simulink model "Test_Tricopter_Model"  (R2015a)
settings: Solver=ode3  SolverMode=SingleTasking  StartTime=0.0  StopTime=20  FixedStep=T_sim  RelTol=1e-3
PreLoadFcn:
  | LoadLibraries
values from neighbouring files (symbols this model uses):
  a = 10.26    [SetupComplete.m]
  A_x = 0.015    [SetupComplete.m]
  A_y = A_x    (= 0.015)    [SetupComplete.m]
  A_z = 0.16    [SetupComplete.m]
  C_d0 = 0.001193    [SetupComplete.m]
  C_x = 1.2    [SetupComplete.m]
  C_y = C_x    (= 1.2)    [SetupComplete.m]
  C_z = 2.2    [SetupComplete.m]
  CG_0 = [0,0,0.02]'    [SetupComplete.m]
  g = 9.81    [SetupComplete.m]
  h = 0.08    [SetupComplete.m]
  h_FA = 0.02    [SetupComplete.m]
  h_M = 0.064    [SetupComplete.m]
  I_BAC_0 = [ Ix,0,Ixz;0,Iy,0;Ixz,0,Iz]    [SetupComplete.m]
  I_prop = 1/4*M_eq*R^2*diag([1,1,2])    [SetupComplete.m]
  I_tube = [1/2*M_tube*R_tube_eq^2,0,  0  ;           0 ,1/3*M_tube*l_arm^2,0;             0  ,0,1/3*M_tube*l_arm^2]    [SetupComplete.m]
  Initial_Omegas = [1;1;1]*Omega_hover    [Run3Copter.m]
  J_FA = I_prop(1,1) + m_prop*h^2  + m_FA*h_FA^2 + m_M*h_M^2    [SetupComplete.m]
  J_T = J_m+1/2*M_eq*R^2    (= 2.000642e-05)    [SetupComplete.m]
  Ki = lqi(LM_4DOF_aug, Q,R)    [robust_controller.m]
  l = 0.3450    (= 0.345)    [NDI_components.m]    (also in SetupComplete.m; robust_controller.m)
  l_arm = 0.264    [SetupComplete.m]
  m = 3.51    [SetupComplete.m]
  m_0 = 2.61    [SetupComplete.m]
  m_FA = 0.02    [SetupComplete.m]
  m_M = 0.300    (= 0.3)    [SetupComplete.m]
  m_prop = 0.02    [SetupComplete.m]
  R = 0.1778    [SetupComplete.m]    (also in robust_controller.m = eye(4))
  rho = 1.15    [SetupComplete.m]
  sigma = b*c/(pi*R)    (= 0.107416159567)    [SetupComplete.m]
  T_sim = 0.01    [Run3Copter.m]
  theta_0 = 0.38397    [SetupComplete.m]
  theta_1 = -0.2967    [SetupComplete.m]
  trim_simplemodel = [0.589627915568 -2.20656039197 0 0.588313336084 0 0 0.588313330414 0 0]    [trimvalues.mat]
  V_4DOF_last = [0.0122475086001 0.00870447045314 -0.0292257707267 -0.0198753669721 -0.00290766514824 -0.0269511839788 0.0344308792695 -0.0305235710433 -0.0274078219028 -0.0329291952852 -0.0272335702183 -0.00643013158961 ... (1500 elements, 50x30)]    [NN_c_weights.mat]
  v_i0 = sqrt( 1/3*m*g/(2*rho*pi*R^2)  )    [SetupComplete.m]
  W_4DOF_last = [0.0132359246225 -0.0402459595001 -0.0221501781133 0.0046881519205 0.0457506835434 0.0464888535199 -0.0342386918322 0.0470592781761 0.0457166948243 -0.00146243512772 0.0300280468889 -0.0358113661373 ... (204 elements, 4x51)]    [NN_c_weights.mat]
undefined symbols (not defined in the file or in its folder): DOWN_0, EAST_0, Motor, NORTH_0, P_0, Prop, Q_0, R_0, sigmatest, U_0, V_0, v_i_adim, Vx_adim, Vz_adim, W_0
undefined symbols (not defined in the file): Initial_Torques, Rotation_sign, Tau_motors
libraries: simulink x61, XXCopter x32, vrlib x26, simulink_extras x6, aerolib6dofsys x3, qcatlib x3, dspinverses x3, lib_controller x2, aerolibtransform2 x2, aerolib6dof2 x1
(part 4 of 10)

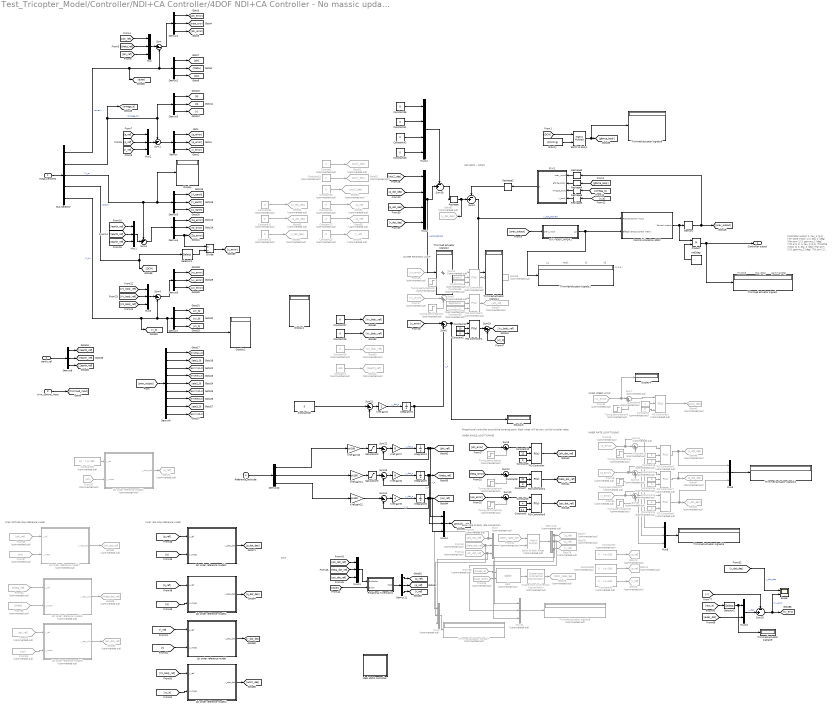
== system Test_Tricopter_Model/Controller/NDI+CA Controller/4DOF NDI+CA Controller - No massic update ==
  note: 16 8
  note: Inner rate loop reference model
  note: w
      | p
      | q
      | r
  note: t1
  note: t2
  note: t3
  note: eta1
  note: OUTER POSITION LOOP
  note: gamma[deg]
  note: eta [deg]
  note: Throttle
  note: Controller output:
      | 1. tau_1 [0-1] (Thr ottle motor 1)
      | 2. eta_1 (deg)  (Pan arm 1)
      | 3. gamma_1 (deg)  (Tilt arm 1)
      |
      | 4. tau_2 [0-1] (Throttle motor 2)
      | 5. eta_2 (deg)  (Pan arm 2)
      | 6. gamma_2 (deg)  (Tilt arm 2)
      |
      | 7. tau_3 [0-1] (Throttle motor 3)
      | 8. eta_3 (deg)  (Pan arm  3)
      | 9. gamma_3 (deg)  (Tilt arm 3)
  note: Proportional controller around the hovering point. Body rates will be very similar to euler rates.
  note: INNER RATE LOOP TUNING
  note: INNER ANGLE LOOP TUNING
  note: INNER SPEED LOOP
  note: NDI 4DOF - WPQR
  note: Euler rate to body rate conversion
  note: Inner attitude loop reference model
  measurements : Inport
  earth_ref : Inport  Port=2
  trim_control_input : Inport  Port=3
  Reference_attitude : Inport  Port=4
  1st order reference model : Subsystem  mask(1st order model reference block){Kref=10, Kb=10, fi=0.25, fc=0.5, Kf=1}
      mask prompts: Kref "1st order reference gain"; Kb "Bandwidth gain"; fi "Integral gain"; fc "Command FF gain"; Kf "Command_dot FF gain"
      mask help:
      | Generates a desired first order derivative of a commanded output taking
      | into account the current measured output.
      | Kref is the gain that determines the first order system between y_ref and
      | y_commanded signals. Ycom/Yref = Kref/(1 + Kref)
      | fi and fc can be defaulted to 0.25 and 0.5 for a critically damped 2nd
      | order response between y_meas and the error signal (y_com - y_meas) considering
      | a perfect dynamic inversion.
      mask Help:
      | Juan Herrero Macias <jn.herrerom@gmail.com>
      | This architecture can be found and explained in Fault-tolerant Flight
      | Control and Guidance Systems, Ducard, Guillaume.
      mask TypeOptions Kref: Kref gain/Gain
      mask TypeOptions Kb: Bandwidth gain/Gain
      mask TypeOptions fi: Integral gain/Gain
      mask TypeOptions fc: Command FF gain/Gain
      mask TypeOptions Kf: Command_dot FF gain/Gain
  1st order reference model1 : Subsystem  mask(1st order model reference block){Kref=8, Kb=16, fi=0.25, fc=0.5, Kf=1}
      mask prompts: Kref "1st order reference gain"; Kb "Bandwidth gain"; fi "Integral gain"; fc "Command FF gain"; Kf "Command_dot FF gain"
      mask help:
      | Generates a desired first order derivative of a commanded output taking
      | into account the current measured output.
      | Kref is the gain that determines the first order system between y_ref and
      | y_commanded signals. Ycom/Yref = Kref/(1 + Kref)
      | fi and fc can be defaulted to 0.25 and 0.5 for a critically damped 2nd
      | order response between y_meas and the error signal (y_com - y_meas) considering
      | a perfect dynamic inversion.
      mask Help:
      | Juan Herrero Macias <jn.herrerom@gmail.com>
      | This architecture can be found and explained in Fault-tolerant Flight
      | Control and Guidance Systems, Ducard, Guillaume.
      mask TypeOptions Kref: Kref gain/Gain
      mask TypeOptions Kb: Bandwidth gain/Gain
      mask TypeOptions fi: Integral gain/Gain
      mask TypeOptions fc: Command FF gain/Gain
      mask TypeOptions Kf: Command_dot FF gain/Gain
  1st order reference model2 : Subsystem  mask(1st order model reference block){Kref=8, Kb=16, fi=0.25, fc=0.5, Kf=1}
      mask prompts: Kref "1st order reference gain"; Kb "Bandwidth gain"; fi "Integral gain"; fc "Command FF gain"; Kf "Command_dot FF gain"
      mask help:
      | Generates a desired first order derivative of a commanded output taking
      | into account the current measured output.
      | Kref is the gain that determines the first order system between y_ref and
      | y_commanded signals. Ycom/Yref = Kref/(1 + Kref)
      | fi and fc can be defaulted to 0.25 and 0.5 for a critically damped 2nd
      | order response between y_meas and the error signal (y_com - y_meas) considering
      | a perfect dynamic inversion.
      mask Help:
      | Juan Herrero Macias <jn.herrerom@gmail.com>
      | This architecture can be found and explained in Fault-tolerant Flight
      | Control and Guidance Systems, Ducard, Guillaume.
      mask TypeOptions Kref: Kref gain/Gain
      mask TypeOptions Kb: Bandwidth gain/Gain
      mask TypeOptions fi: Integral gain/Gain
      mask TypeOptions fc: Command FF gain/Gain
      mask TypeOptions Kf: Command_dot FF gain/Gain
  1st order reference model3 : Subsystem  Commented=on  mask(1st order model reference block){Kref=2, Kb=2, fi=0.25, fc=0, Kf=0}
      mask prompts: Kref "1st order reference gain"; Kb "Bandwidth gain"; fi "Integral gain"; fc "Command FF gain"; Kf "Command_dot FF gain"
      mask help:
      | Generates a desired first order derivative of a commanded output taking
      | into account the current measured output.
      | Kref is the gain that determines the first order system between y_ref and
      | y_commanded signals. Ycom/Yref = Kref/(1 + Kref)
      | fi and fc can be defaulted to 0.25 and 0.5 for a critically damped 2nd
      | order response between y_meas and the error signal (y_com - y_meas) considering
      | a perfect dynamic inversion.
      mask Help:
      | Juan Herrero Macias <jn.herrerom@gmail.com>
      | This architecture can be found and explained in Fault-tolerant Flight
      | Control and Guidance Systems, Ducard, Guillaume.
      mask TypeOptions Kref: Kref gain/Gain
      mask TypeOptions Kb: Bandwidth gain/Gain
      mask TypeOptions fi: Integral gain/Gain
      mask TypeOptions fc: Command FF gain/Gain
      mask TypeOptions Kf: Command_dot FF gain/Gain
  1st order reference model4 : Subsystem  mask(1st order model reference block){Kref=4, Kb=8, fi=0.25, fc=0.5, Kf=1}
      mask prompts: Kref "1st order reference gain"; Kb "Bandwidth gain"; fi "Integral gain"; fc "Command FF gain"; Kf "Command_dot FF gain"
      mask help:
      | Generates a desired first order derivative of a commanded output taking
      | into account the current measured output.
      | Kref is the gain that determines the first order system between y_ref and
      | y_commanded signals. Ycom/Yref = Kref/(1 + Kref)
      | fi and fc can be defaulted to 0.25 and 0.5 for a critically damped 2nd
      | order response between y_meas and the error signal (y_com - y_meas) considering
      | a perfect dynamic inversion.
      mask Help:
      | Juan Herrero Macias <jn.herrerom@gmail.com>
      | This architecture can be found and explained in Fault-tolerant Flight
      | Control and Guidance Systems, Ducard, Guillaume.
      mask TypeOptions Kref: Kref gain/Gain
      mask TypeOptions Kb: Bandwidth gain/Gain
      mask TypeOptions fi: Integral gain/Gain
      mask TypeOptions fc: Command FF gain/Gain
      mask TypeOptions Kf: Command_dot FF gain/Gain
  1st order reference model5 : Subsystem  Commented=on  mask(1st order model reference block){Kref=8, Kb=4, fi=0.25, fc=0.5, Kf=1}
      mask prompts: Kref "1st order reference gain"; Kb "Bandwidth gain"; fi "Integral gain"; fc "Command FF gain"; Kf "Command_dot FF gain"
      mask help:
      | Generates a desired first order derivative of a commanded output taking
      | into account the current measured output.
      | Kref is the gain that determines the first order system between y_ref and
      | y_commanded signals. Ycom/Yref = Kref/(1 + Kref)
      | fi and fc can be defaulted to 0.25 and 0.5 for a critically damped 2nd
      | order response between y_meas and the error signal (y_com - y_meas) considering
      | a perfect dynamic inversion.
      mask Help:
      | Juan Herrero Macias <jn.herrerom@gmail.com>
      | This architecture can be found and explained in Fault-tolerant Flight
      | Control and Guidance Systems, Ducard, Guillaume.
      mask TypeOptions Kref: Kref gain/Gain
      mask TypeOptions Kb: Bandwidth gain/Gain
      mask TypeOptions fi: Integral gain/Gain
      mask TypeOptions fc: Command FF gain/Gain
      mask TypeOptions Kf: Command_dot FF gain/Gain
  1st order reference model6 : Subsystem  Commented=on  mask(1st order model reference block){Kref=2, Kb=4, fi=0.25, fc=0.5, Kf=1}
      mask prompts: Kref "1st order reference gain"; Kb "Bandwidth gain"; fi "Integral gain"; fc "Command FF gain"; Kf "Command_dot FF gain"
      mask help:
      | Generates a desired first order derivative of a commanded output taking
      | into account the current measured output.
      | Kref is the gain that determines the first order system between y_ref and
      | y_commanded signals. Ycom/Yref = Kref/(1 + Kref)
      | fi and fc can be defaulted to 0.25 and 0.5 for a critically damped 2nd
      | order response between y_meas and the error signal (y_com - y_meas) considering
      | a perfect dynamic inversion.
      mask Help:
      | Juan Herrero Macias <jn.herrerom@gmail.com>
      | This architecture can be found and explained in Fault-tolerant Flight
      | Control and Guidance Systems, Ducard, Guillaume.
      mask TypeOptions Kref: Kref gain/Gain
      mask TypeOptions Kb: Bandwidth gain/Gain
      mask TypeOptions fi: Integral gain/Gain
      mask TypeOptions fc: Command FF gain/Gain
      mask TypeOptions Kf: Command_dot FF gain/Gain
  1st order reference model7 : Subsystem  Commented=on  mask(1st order model reference block){Kref=8, Kb=4, fi=0.25, fc=0.5, Kf=1}
      mask prompts: Kref "1st order reference gain"; Kb "Bandwidth gain"; fi "Integral gain"; fc "Command FF gain"; Kf "Command_dot FF gain"
      mask help:
      | Generates a desired first order derivative of a commanded output taking
      | into account the current measured output.
      | Kref is the gain that determines the first order system between y_ref and
      | y_commanded signals. Ycom/Yref = Kref/(1 + Kref)
      | fi and fc can be defaulted to 0.25 and 0.5 for a critically damped 2nd
      | order response between y_meas and the error signal (y_com - y_meas) considering
      | a perfect dynamic inversion.
      mask Help:
      | Juan Herrero Macias <jn.herrerom@gmail.com>
      | This architecture can be found and explained in Fault-tolerant Flight
      | Control and Guidance Systems, Ducard, Guillaume.
      mask TypeOptions Kref: Kref gain/Gain
      mask TypeOptions Kb: Bandwidth gain/Gain
      mask TypeOptions fi: Integral gain/Gain
      mask TypeOptions fc: Command FF gain/Gain
      mask TypeOptions Kf: Command_dot FF gain/Gain
  Bus Selector : BusSelector  OutputSignals=euler,omega_b,X_e,DCM,V_b
  Constant{,3,14,16,18..23,29..33,35} (16 alike) : Constant  Commented=on  Value=0
  Constant1 : Constant  Commented=on  Value=-100
  Constant10 : Constant  Value=12
  Constant11 : Constant  Value=10
  Constant12 : Constant  Commented=on  Value=deg2rad(1)
  Constant13 : Constant  Commented=on  Value=6
  Constant15 : Constant  Commented=on  Value=5
  Constant17 : Constant  Commented=on  Value=6
  Constant{2,27..28,36,41..43,45} (8 alike) : Constant  Value=0
  Constant34 : Constant  Commented=on  Value=deg2rad(1)
  Constant37 : Constant  Commented=on  Value="0     * pi /180"
  Constant38 : Constant  Commented=on  Value="10     * pi /180"
  Constant39 : Constant  Commented=on  Value="0     * pi /180"
  Constant4 : Constant  Commented=on
  Constant40 : Constant  Commented=on  Value="0     * pi /180"
  Constant5 : Constant  Value=0.4
  Constant6 : Constant  Value=4
  Constant7 : Constant  Value=3
  Constant8 : Constant  Value=12
  Constant9 : Constant  Value=3
  Control Allocation 4DOF : Subsystem  Variant=on  OverrideUsingVariant=Variant1
  Demux{,1..8,11,13} (11 alike) : Demux  Outputs=3
  Demux10 : Demux  Commented=on  Outputs=3
  Demux9 : Demux  Outputs=9
  Display{,1..4} (5 alike) : Display
  Divide : Product  Inputs=*/
  Earth to body Rates : Product  Commented=on  Multiplication=Matrix(*)
  Earth to body1 : Product  Multiplication=Matrix(*)
  F(X)1 : MATLAB Function  TreatAsAtomicUnit=on
  From17 : From  Commented=on  GotoTag=vy_error
  From18 : From  Commented=on  GotoTag=vx_error
  From21 : From  Commented=on  GotoTag=vz_error
  From25 : From  Commented=on  GotoTag=quat_euler
  From26 : From  Commented=on  GotoTag=p_error
  From28 : From  Commented=on  GotoTag=q_error
  From29 : From  Commented=on  GotoTag=r_error
  From35 : From  Commented=on  GotoTag=phi
  From36 : From  Commented=on  GotoTag=omega_b
  From37 : From  Commented=on  GotoTag=phi_dot_ref
  From40 : From  Commented=on  GotoTag=theta_dot_ref
  From41 : From  Commented=on  GotoTag=psi_dot_ref
  From42 : From  Commented=on  GotoTag=DCM_rates_be
  From54 : From  Commented=on  GotoTag=theta_ref
  From55 : From  Commented=on  GotoTag=theta
  From56 : From  Commented=on  GotoTag=phi_ref
  From57 : From  Commented=on  GotoTag=phi
  From58 : From  Commented=on  GotoTag=psi_ref
  From59 : From  Commented=on  GotoTag=psi
  G(X) 4DOF_WPQR1 : MATLAB Function  TreatAsAtomicUnit=on
  Goto40 : Goto  Commented=on  GotoTag=Zearth_ref
  Goto41 : Goto  Commented=on  GotoTag=accZ_des
  Goto46 : Goto  Commented=on  GotoTag=p_dot_des
  Goto47 : Goto  Commented=on  GotoTag=q_dot_des
  Goto48 : Goto  Commented=on  GotoTag=r_dot_des
  Goto51 : Goto  Commented=on  GotoTag=accX_des
  Goto52 : Goto  Commented=on  GotoTag=accY_des
  Goto53 : Goto  Commented=on  GotoTag=accZ_des
  Goto{54,72..73,77} (4 alike) : Goto  Commented=on  GotoTag=p_ref
  Goto55 : Goto  Commented=on  GotoTag=q_ref
  Goto56 : Goto  Commented=on  GotoTag=r_ref
  Goto63 : Goto  Commented=on  GotoTag=Vz_body_ref
  Goto64 : Goto  Commented=on  GotoTag=p_dot_des
  Goto65 : Goto  Commented=on  GotoTag=q_dot_des
  Goto66 : Goto  Commented=on  GotoTag=r_dot_des
  Goto67 : Goto  Commented=on  GotoTag=phi_ref
  Goto68 : Goto  Commented=on  GotoTag=theta_ref
  Goto74 : Goto  Commented=on  GotoTag=q_ref
  Goto75 : Goto  Commented=on  GotoTag=r_ref
  Goto76 : Goto  Commented=on  GotoTag=DCM_rates_be
  Goto78 : Goto  Commented=on  GotoTag=q_ref
  Goto79 : Goto  Commented=on  GotoTag=r_ref
  Goto87 : Goto  Commented=on  GotoTag=y_dot_des
  Goto89 : Goto  Commented=on  GotoTag=theta_dot_ref
  Goto90 : Goto  Commented=on  GotoTag=phi_dot_ref
  Goto91 : Goto  Commented=on  GotoTag=psi_dot_ref
  Gravity : Constant  Value=[0;0;m*g]
  Ideal 4DOF controller : Subsystem
  Integrator{3..6} (4 alike) : Integrator
  Kref gain10 : Gain  Gain=pi/180
  Kref gain11 : Gain  Gain=pi/180
  Kref gain12 : Gain  Gain=pi/180
  Kref gain3 : Gain
  Kref gain7 : Gain  Gain=6
  Kref gain8 : Gain  Gain=6
  Kref gain9 : Gain  Gain=4
  Memory : Memory  X0=[0,0,0,0,0,0,0,0,0]  LinearizeAsDelay=on
  Mux{,1..3,5,8,11,14} (8 alike) : Mux  Inputs=3
  Mux10 : Mux  Commented=on  Inputs=3
  Mux12 : Mux
  Mux13 : Mux  Inputs=2
  Mux4 : Mux
  Mux7 : Mux  Commented=on  Inputs=3
  Mux9 : Mux  Commented=on  Inputs=3
  PID Controller{,1,4..5} (4 alike) : simulink/Continuous/PID Controller  Controller=PI  TimeDomain=Continuous-time  SampleTime=-1  IntegratorMethod=Forward Euler  FilterMethod=Forward Euler  Form=Parallel  UseFilter=on  ControllerParametersSource=external  P=1  I=1  D=0  N=100  InitialConditionSource=internal  InitialConditionForIntegrator=0  InitialConditionForFilter=0  ExternalReset=none  LimitOutput=off  UpperSaturationLimit=inf  LowerSaturationLimit=-inf  LinearizeAsGain=on  AntiWindupMode=none  Kb=1  TrackingMode=off  Kt=1  PParamMin=[]  PParamMax=[]  IParamMin=[]  IParamMax=[]  DParamMin=[]  DParamMax=[]  NParamMin=[]  NParamMax=[]  KbParamMin=[]  KbParamMax=[]  KtParamMin=[]  KtParamMax=[]  POutMin=[]  POutMax=[]  IOutMin=[]  IOutMax=[]  DOutMin=[]  DOutMax=[]  NOutMin=[]  NOutMax=[]  KbOutMin=[]  KbOutMax=[]  KtOutMin=[]  KtOutMax=[]  IntegratorOutMin=[]  IntegratorOutMax=[]  FilterOutMin=[]  FilterOutMax=[]  SumOutMin=[]  SumOutMax=[]  SumI1OutMin=[]  SumI1OutMax=[]  SumI2OutMin=[]  SumI2OutMax=[]  SumI3OutMin=[]  SumI3OutMax=[]  SumDOutMin=[]  SumDOutMax=[]  SaturationOutMin=[]  SaturationOutMax=[]  IntegratorContinuousStateAttributes=''  IntegratorStateMustResolveToSignalObject=off  IntegratorRTWStateStorageClass=Auto  FilterContinuousStateAttributes=''  FilterStateMustResolveToSignalObject=off  FilterRTWStateStorageClass=Auto  DifferentiatorICPrevScaledInput=0  DifferentiatorOutMin=[]  DifferentiatorOutMax=[]
  PID Controller{2..3,8..9} (4 alike) : simulink/Continuous/PID Controller  Commented=on  Controller=PI  TimeDomain=Continuous-time  SampleTime=-1  IntegratorMethod=Forward Euler  FilterMethod=Forward Euler  Form=Parallel  UseFilter=on  ControllerParametersSource=external  P=1  I=1  D=0  N=100  InitialConditionSource=internal  InitialConditionForIntegrator=0  InitialConditionForFilter=0  ExternalReset=none  LimitOutput=off  UpperSaturationLimit=inf  LowerSaturationLimit=-inf  LinearizeAsGain=on  AntiWindupMode=none  Kb=1  TrackingMode=off  Kt=1  PParamMin=[]  PParamMax=[]  IParamMin=[]  IParamMax=[]  DParamMin=[]  DParamMax=[]  NParamMin=[]  NParamMax=[]  KbParamMin=[]  KbParamMax=[]  KtParamMin=[]  KtParamMax=[]  POutMin=[]  POutMax=[]  IOutMin=[]  IOutMax=[]  DOutMin=[]  DOutMax=[]  NOutMin=[]  NOutMax=[]  KbOutMin=[]  KbOutMax=[]  KtOutMin=[]  KtOutMax=[]  IntegratorOutMin=[]  IntegratorOutMax=[]  FilterOutMin=[]  FilterOutMax=[]  SumOutMin=[]  SumOutMax=[]  SumI1OutMin=[]  SumI1OutMax=[]  SumI2OutMin=[]  SumI2OutMax=[]  SumI3OutMin=[]  SumI3OutMax=[]  SumDOutMin=[]  SumDOutMax=[]  SaturationOutMin=[]  SaturationOutMax=[]  IntegratorContinuousStateAttributes=''  IntegratorStateMustResolveToSignalObject=off  IntegratorRTWStateStorageClass=Auto  FilterContinuousStateAttributes=''  FilterStateMustResolveToSignalObject=off  FilterRTWStateStorageClass=Auto  DifferentiatorICPrevScaledInput=0  DifferentiatorOutMin=[]  DifferentiatorOutMax=[]
  PID Controller6 : simulink/Continuous/PID Controller  Commented=on  Controller=PI  TimeDomain=Continuous-time  SampleTime=-1  IntegratorMethod=Forward Euler  FilterMethod=Forward Euler  Form=Parallel  UseFilter=on  ControllerParametersSource=external  P=121.80671459326  I=327.532586687046  D=0  N=100  InitialConditionSource=internal  InitialConditionForIntegrator=0  InitialConditionForFilter=0  ExternalReset=none  LimitOutput=off  UpperSaturationLimit=inf  LowerSaturationLimit=-inf  LinearizeAsGain=on  AntiWindupMode=none  Kb=1  TrackingMode=off  Kt=1  PParamMin=[]  PParamMax=[]  IParamMin=[]  IParamMax=[]  DParamMin=[]  DParamMax=[]  NParamMin=[]  NParamMax=[]  KbParamMin=[]  KbParamMax=[]  KtParamMin=[]  KtParamMax=[]  POutMin=[]  POutMax=[]  IOutMin=[]  IOutMax=[]  DOutMin=[]  DOutMax=[]  NOutMin=[]  NOutMax=[]  KbOutMin=[]  KbOutMax=[]  KtOutMin=[]  KtOutMax=[]  IntegratorOutMin=[]  IntegratorOutMax=[]  FilterOutMin=[]  FilterOutMax=[]  SumOutMin=[]  SumOutMax=[]  SumI1OutMin=[]  SumI1OutMax=[]  SumI2OutMin=[]  SumI2OutMax=[]  SumI3OutMin=[]  SumI3OutMax=[]  SumDOutMin=[]  SumDOutMax=[]  SaturationOutMin=[]  SaturationOutMax=[]  IntegratorContinuousStateAttributes=''  IntegratorStateMustResolveToSignalObject=off  IntegratorRTWStateStorageClass=Auto  FilterContinuousStateAttributes=''  FilterStateMustResolveToSignalObject=off  FilterRTWStateStorageClass=Auto  DifferentiatorICPrevScaledInput=0  DifferentiatorOutMin=[]  DifferentiatorOutMax=[]
  PID Controller7 : simulink/Continuous/PID Controller  Commented=on  Controller=PI  TimeDomain=Continuous-time  SampleTime=-1  IntegratorMethod=Forward Euler  FilterMethod=Forward Euler  Form=Parallel  UseFilter=on  ControllerParametersSource=external  P=244.169484479421  I=1759.80724182952  D=0  N=100  InitialConditionSource=internal  InitialConditionForIntegrator=0  InitialConditionForFilter=0  ExternalReset=none  LimitOutput=off  UpperSaturationLimit=inf  LowerSaturationLimit=-inf  LinearizeAsGain=on  AntiWindupMode=none  Kb=1  TrackingMode=off  Kt=1  PParamMin=[]  PParamMax=[]  IParamMin=[]  IParamMax=[]  DParamMin=[]  DParamMax=[]  NParamMin=[]  NParamMax=[]  KbParamMin=[]  KbParamMax=[]  KtParamMin=[]  KtParamMax=[]  POutMin=[]  POutMax=[]  IOutMin=[]  IOutMax=[]  DOutMin=[]  DOutMax=[]  NOutMin=[]  NOutMax=[]  KbOutMin=[]  KbOutMax=[]  KtOutMin=[]  KtOutMax=[]  IntegratorOutMin=[]  IntegratorOutMax=[]  FilterOutMin=[]  FilterOutMax=[]  SumOutMin=[]  SumOutMax=[]  SumI1OutMin=[]  SumI1OutMax=[]  SumI2OutMin=[]  SumI2OutMax=[]  SumI3OutMin=[]  SumI3OutMax=[]  SumDOutMin=[]  SumDOutMax=[]  SaturationOutMin=[]  SaturationOutMax=[]  IntegratorContinuousStateAttributes=''  IntegratorStateMustResolveToSignalObject=off  IntegratorRTWStateStorageClass=Auto  FilterContinuousStateAttributes=''  FilterStateMustResolveToSignalObject=off  FilterRTWStateStorageClass=Auto  DifferentiatorICPrevScaledInput=0  DifferentiatorOutMin=[]  DifferentiatorOutMax=[]
  Product : Product
  Quaternions to Direction Cosine Matrix : aerolibtransform2/Quaternions to  Direction Cosine Matrix  Commented=on
  Reshape : Reshape  OutputDimensionality=Column vector (2-D)
  Reshape2 : Reshape  OutputDimensionality=Column vector (2-D)  OutputDimensions=[6,1]
  Reshape{3..6} (4 alike) : Reshape  OutputDimensions=[6,1]
  Rotational Kinematics : MATLAB Function  TreatAsAtomicUnit=on
  Saturation2 : Saturate  UpperLimit=30  LowerLimit=-30
  Saturation3 : Saturate  UpperLimit=30  LowerLimit=-30
  Scope : Scope  NumInputPorts=2
      settings: ShowLegends=on  YMin=-5~-20  YMax=15~20
  Selector1 : Selector  NumberOfDimensions=2  InputPortWidth=[9]  IndexOptions=Index vector (dialog),Index vector (dialog)  Indices=3,3  OutputSizes=1,1
  Selector2 : Selector  InputPortWidth=3  Indices=[3]
  Sum{,4,21..24} (6 alike) : Sum  Inputs=|+-
  Sum{1..3,18,20} (5 alike) : Sum  Inputs=-+|
  Sum{5,9..10,12,19} (5 alike) : Sum  Inputs=|++
  Sum{6..8,11,13..14} (6 alike) : Sum  Commented=on  Inputs=|++
  Trimmed actuator signals{,1..6,9} (8 alike) : Display
  Trimmed actuator signals7 : Display  Commented=on
  Trimmed actuator signals8 : Display  Commented=on
  Tuning perturbation{,5..6,8} (4 alike) : Step  Commented=on  Time=20  After=3*pi/180  SampleTime=0
  Tuning perturbation2 : Step  Commented=on  Time=20  SampleTime=0
  Tuning perturbation3 : Step  Commented=on  Time=20  SampleTime=0
  Tuning perturbation4 : Step  Commented=on  Time=20  After=-3*pi/180  SampleTime=0
  Tuning perturbation7 : Step  Commented=on  Time=20  After=-3*pi/180  SampleTime=0
  Tuning perturbation9 : Step  Commented=on  Time=20  SampleTime=0
  qdot : aerolib6dofsys/DCM & Euler Angles (Quaternion)/qdot  Commented=on
  rad2deg : Constant  Value=[1, 180/pi, 0,1,0, 0, 1, 0,0]
  Controller output : Outport
  tag scope: attitude_com=global, inv_error=global
  wires:
  [vz_b] -> Sum19/2
  Sum19/1 -> [Vz_body_ref]
  PID Controller1/1 -> Sum19/1
  Selector1/1 -> Divide/2
  Demux4/3 -> [Ze_error], Divide/1
  Sum18/1 -> Reshape/1
  Mux12/1 -> Sum18/1
  Constant43/1 -> Mux12/4
  Constant42/1 -> Mux12/3
  Constant41/1 -> Mux12/2
  Constant36/1 -> Mux12/1
  Mux11/1 -> Rotational Kinematics/1(Eulerdot)
  [psi_dot_ref] -> Mux11/3
  [theta_dot_ref] -> Mux11/2
  [phi_dot_ref] -> Mux11/1
  Rotational Kinematics/1(PQR) -> Demux11/1
  Demux11/3 -> [r_ref]
  Demux11/2 -> [q_ref]
  Demux11/1 -> [p_ref]
  [euler] -> Rotational Kinematics/2(Euler)
  Mux10/1 -> Trimmed actuator signals8/1
  Demux10/3 -> Mux10/3, Goto79/1
  Demux10/2 -> Goto78/1, Mux10/2
  Demux10/1 -> Goto77/1, Mux10/1
  Mux9/1 -> Trimmed actuator signals7/1
  From41/1 -> Mux7/3, Mux9/3
  From40/1 -> Mux7/2, Mux9/2
  From37/1 -> Mux7/1, Mux9/1
  Quaternions to Direction Cosine Matrix/1 -> Goto76/1
  From25/1 -> qdot/2
  qdot/1 -> Quaternions to Direction Cosine Matrix/1
  From36/1 -> qdot/1
  Earth to body Rates/1 -> Demux10/1
  From42/1 -> Earth to body Rates/1
  Mux7/1 -> Earth to body Rates/2
  Divide/1 -> [z_error]
  Constant40/1 -> Goto75/1
  Constant39/1 -> Goto74/1
  Constant37/1 -> Goto73/1
  Constant14/1 -> PID Controller8/3
  Constant18/1 -> PID Controller6/3
  Constant38/1 -> 1st order reference model3/1(y_ref)
  1st order reference model3/1(y_des_dot) -> Goto72/1
  From35/1 -> 1st order reference model3/2(y_meas)
  [p_ref] -> 1st order reference model2/1(y_ref)
  1st order reference model2/1(y_des_dot) -> [p_dot_des]
  [p] -> 1st order reference model2/2(y_meas)
  G(X) 4DOF_WPQR1/1(gx) -> Control Allocation 4DOF/2(Effectiveness control matrix), Trimmed actuator signals1/1
  PID Controller9/1 -> Goto68/1
  Tuning perturbation9/1 -> Sum11/2
  From18/1 -> Sum11/1
  Sum11/1 -> PID Controller9/1
  Constant35/1 -> PID Controller9/3
  Constant34/1 -> PID Controller9/2
  PID Controller3/1 -> Goto67/1
  Tuning perturbation2/1 -> Sum6/2
  From17/1 -> Sum6/1
  Sum6/1 -> PID Controller3/1
  Constant33/1 -> PID Controller3/3
  Constant12/1 -> PID Controller3/2
  [z_error] -> Sum5/1
  Sum5/1 -> PID Controller1/1, Display3/1
  Constant2/1 -> PID Controller1/3
  Constant11/1 -> PID Controller1/2
  Constant1/1 -> Goto40/1
  [r_dot_des] -> Mux4/4
  [q_dot_des] -> Mux4/3
  [p_dot_des] -> Mux4/2
  [accZ_des] -> Mux4/1
  [prev_output] -> G(X) 4DOF_WPQR1/1(prev_input)
  Control Allocation 4DOF/1(Control output) -> Memory/1, Product/1
  Sum2/1 -> Control Allocation 4DOF/1(Pseudocontrol input), Trimmed actuator signals4/1  "y_dot_desired"
  Constant13/1 -> PID Controller6/2
  Sum3/1 -> Demux4/1
  Constant32/1 -> Goto66/1
  Constant31/1 -> Goto65/1
  Constant30/1 -> Goto64/1
  Memory/1 -> [prev_output], Reshape3/1
  [DCM] -> Earth to body1/1
  Mux8/1 -> Trimmed actuator signals5/1
  From29/1 -> Sum8/1, Mux8/3
  From28/1 -> Sum13/1, Mux8/2
  From26/1 -> Sum14/1, Mux8/1
  [psi_error] -> Sum10/1
  [theta_error] -> Sum12/1
  [phi_error] -> Sum9/1
  Constant29/1 -> Goto63/1
  Constant28/1 -> [Vy_body_ref]
  Constant27/1 -> [Vx_body_ref]
  PID Controller2/1 -> Goto41/1
  Mux5/1 -> Trimmed actuator signals3/1
  1st order reference model/1(y_des_dot) -> [r_dot_des]
  [r] -> 1st order reference model/2(y_meas)
  [r_ref] -> 1st order reference model/1(y_ref)
  rad2deg/1 -> Product/2
  Product/1 -> Controller output/1, Trimmed actuator signals/1
  Constant23/1 -> Goto56/1
  Constant22/1 -> Goto55/1
  Constant21/1 -> Goto54/1
  Constant20/1 -> Goto53/1
  Constant19/1 -> Goto52/1
  Constant/1 -> Goto51/1
  [v_b] -> Reshape6/1
  Reshape6/1 -> F(X)1/4(v_body)
  Reshape5/1 -> F(X)1/3(omega_body)
  Reshape4/1 -> F(X)1/2(gforce_body)
  [omega_b] -> Reshape5/1
  Reshape3/1 -> F(X)1/1(prev_input)
  Reshape2/1 -> Sum2/1
  Reshape/1 -> Goto87/1, Sum2/2
  Mux4/1 -> Sum18/2, Trimmed actuator signals2/1  "y_dot_desired"
  Tuning perturbation7/1 -> Sum13/2
  Tuning perturbation6/1 -> Sum14/2
  Tuning perturbation8/1 -> Sum8/2
  Sum13/1 -> PID Controller7/1
  Sum8/1 -> PID Controller8/1
  Sum14/1 -> PID Controller6/1
  Constant16/1 -> PID Controller7/3
  Constant17/1 -> PID Controller7/2
  Constant15/1 -> PID Controller8/2
  PID Controller8/1 -> Goto48/1, Mux5/3
  PID Controller7/1 -> Goto47/1, Mux5/2
  PID Controller6/1 -> Goto46/1, Mux5/1
  Tuning perturbation4/1 -> Sum12/2
  Tuning perturbation/1 -> Sum9/2
  Tuning perturbation5/1 -> Sum10/2
  Sum12/1 -> PID Controller4/1
  Sum10/1 -> PID Controller5/1
  Sum9/1 -> PID Controller/1
  Constant7/1 -> PID Controller4/3
  Constant9/1 -> PID Controller/3
  Constant10/1 -> PID Controller/2
  Constant8/1 -> PID Controller4/2
  Constant5/1 -> PID Controller5/3
  Constant6/1 -> PID Controller5/2
  PID Controller5/1 -> [psi_dot_ref]
  PID Controller4/1 -> [theta_dot_ref]
  PID Controller/1 -> [phi_dot_ref]
  Tuning perturbation3/1 -> Sum7/2
  From21/1 -> Sum7/1, Display4/1
  Sum7/1 -> PID Controller2/1
  Constant3/1 -> PID Controller2/3
  Constant4/1 -> PID Controller2/2
  [gforce_body] -> Reshape4/1
  Earth to body1/1 -> [gforce_body], Trimmed actuator signals6/1
  Gravity/1 -> Earth to body1/2
  F(X)1/1(fx) -> Reshape2/1
  Mux/1 -> Sum/1
  Demux3/3 -> [r]
  Demux3/2 -> [q]
  Demux3/1 -> [p]
  Demux2/1 -> [phi]
  Demux2/2 -> [theta]
  Demux2/3 -> [psi]
  measurements/1 -> Bus Selector/1
  Bus Selector/1 -> Demux2/1, Sum/2, [euler]  "<euler>"
  Bus Selector/2 -> Demux3/1, Sum1/1, [omega_b]  "<omega_b>"
  Sum1/1 -> Demux/1
  Sum/1 -> Demux1/1
  Demux/3 -> [r_error]
  Demux/2 -> [q_error]
  Demux/1 -> [p_error]
  Demux1/1 -> [phi_error]
  Demux1/2 -> [theta_error]
  Demux1/3 -> [psi_error]
  trim_control_input/1 -> [trimmed_input]
  [theta_ref] -> Mux/2
  [phi_ref] -> Mux/1
  [psi_ref] -> Mux/3
  Mux2/1 -> Sum1/2
  [q_ref] -> Mux2/2
  [p_ref] -> Mux2/1
  [r_ref] -> Mux2/3
  Bus Selector/3 -> Sum3/1, Demux5/1, Display/1  "<X_e>"
  Demux5/3 -> [Z_earth]
  Demux5/2 -> [Y_earth]
  Demux5/1 -> [X_earth]
  Demux4/2 -> [Ye_error]
  Demux4/1 -> [Xe_error]
  Mux1/1 -> Sum3/2
  [Yearth_ref] -> Mux1/2
  [Xearth_ref] -> Mux1/1
  [Zearth_ref] -> Mux1/3
  Mux3/1 -> Sum4/1
  Demux7/1 -> [vx_b]
  Demux7/2 -> [vy_b]
  Demux7/3 -> [vz_b]
  Bus Selector/5 -> Demux7/1, Display2/1, Sum4/2, [v_b]  "<V_b>"
  Sum4/1 -> Demux6/1
  Demux6/1 -> [vx_error]
  Demux6/2 -> [vy_error]
  Demux6/3 -> [vz_error]
  [Vy_body_ref] -> Mux3/2
  [Vx_body_ref] -> Mux3/1
  [Vz_body_ref] -> Mux3/3
  Bus Selector/4 -> Selector1/1, [DCM]  "<DCM>"
  Demux8/3 -> [Zearth_ref]
  Demux8/2 -> [Yearth_ref]
  Demux8/1 -> [Xearth_ref]
  earth_ref/1 -> Demux8/1
  [prev_output] -> Demux9/1
  Demux9/1 -> [throttle1_0]
  Demux9/2 -> [eta1_0]
  Demux9/3 -> [gamma1_0]
  Demux9/4 -> [throttle2_0]
  Demux9/5 -> [eta2_0]
  Demux9/6 -> [gamma2_0]
  Demux9/7 -> [throttle3_0]
  Demux9/8 -> [eta3_0]
  Demux9/9 -> [gamma3_0]
  [Vz_body_ref] -> 1st order reference model4/1(y_ref)
  1st order reference model4/1(y_des_dot) -> [accZ_des]
  [vz_b] -> 1st order reference model4/2(y_meas)
  Sum21/1 -> Kref gain3/1
  Kref gain3/1 -> Integrator3/1  "y_dot_c"
  Integrator3/1 -> Sum5/2, Sum21/2  "y_c"
  Constant45/1 -> Sum21/1
  [euler_dot] -> Mux13/2
  [acc_b] -> Selector2/1
  [y_dot_des] -> Scope/1  "y_dot_des"
  Mux13/1 -> Sum20/2  "y_dot"
  [v] -> Sum20/1
  Sum20/1 -> [inv_error], Scope/2  "inv_error"
  Selector2/1 -> Trimmed actuator signals9/1, Mux13/1
  From56/1 -> 1st order reference model7/1(y_ref)
  1st order reference model7/1(y_des_dot) -> Goto90/1
  From57/1 -> 1st order reference model7/2(y_meas)
  1st order reference model5/1(y_des_dot) -> Goto89/1
  From55/1 -> 1st order reference model5/2(y_meas)
  From54/1 -> 1st order reference model5/1(y_ref)
  From58/1 -> 1st order reference model6/1(y_ref)
  1st order reference model6/1(y_des_dot) -> Goto91/1
  From59/1 -> 1st order reference model6/2(y_meas)
  [q_ref] -> 1st order reference model1/1(y_ref)
  1st order reference model1/1(y_des_dot) -> [q_dot_des]
  [q] -> 1st order reference model1/2(y_meas)
  Saturation3/1 -> Sum23/1
  Saturation2/1 -> Sum22/1
  Sum24/1 -> Kref gain9/1
  Kref gain9/1 -> Integrator6/1  "y_dot_c"
  Integrator6/1 -> Mux14/3, [psi_ref], Sum24/2  "y_c"
  Sum23/1 -> Kref gain8/1
  Kref gain8/1 -> Integrator5/1  "y_dot_c"
  Integrator5/1 -> Sum23/2, Mux14/2, [theta_ref]  "y_c"
  Sum22/1 -> Kref gain7/1
  Kref gain7/1 -> Integrator4/1  "y_dot_c"
  Integrator4/1 -> Mux14/1, [phi_ref], Sum22/2  "y_c"
  Kref gain10/1 -> Saturation2/1
  Kref gain11/1 -> Saturation3/1
  Kref gain12/1 -> Sum24/1
  Reference_attitude/1 -> Demux13/1
  Demux13/1 -> Kref gain10/1
  Demux13/2 -> Kref gain11/1
  Demux13/3 -> Kref gain12/1
  Mux14/1 -> [attitude_com]

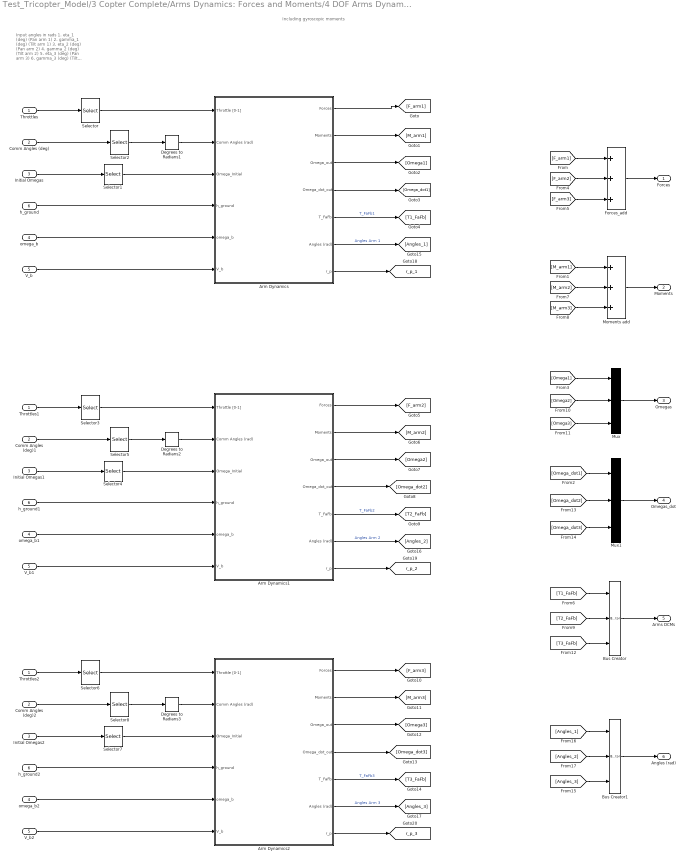
== system Test_Tricopter_Model/3 Copter Complete/Arms Dynamics: Forces and Moments/4 DOF Arms Dynamics: Forces and Moments1/4 DOF Arms Dynamics: Forces and Moments1 ==
  note: Including gyroscopic moments
  note: Input angles in rads
      |
      | 1. eta_1 (deg)  (Pan arm 1)
      | 2. gamma_1 (deg)  (Tilt arm 1)
      |
      | 3. eta_2 (deg)  (Pan arm 2)
      | 4. gamma_2 (deg)  (Tilt arm 2)
      |
      | 5. eta_3 (deg)  (Pan arm  3)
      | 6. gamma_3 (deg)  (Tilt arm 3)
  Throttles : Inport
  Comm Angles (deg) : Inport  Port=2
  Initial Omegas : Inport  Port=3
  omega_b : Inport  Port=4
  V_b : Inport  Port=5
  h_ground : Inport  Port=6
  Arm Dynamics : Subsystem  AncestorBlock=XXCopter/Arm Dynamics  TreatAsAtomicUnit=on  mask(Arm dynamics, kinematics, forces and moments){Rot_sign=Rotation_sign(1), tau=Tau_motors, arm_hub_pos=l*[1;0;0], arm_axis=[l_arm;0;0], arm_num=1, eta_dir=[1;0;0], gamma_dir=[0;1;0], J_T=J_T, J_FA=J_FA, h=h, Torq_ini=Initial_Torques(1), Omega_ini=Initial_Omegas(1), init_eta=0, init_gamma=0, omega_n=35, xi=1.45, c=0.01}
      mask prompts: Rot_sign "Rotation sign"; tau "Tau motors"; arm_hub_pos "Arm Hub position"; arm_axis "Arm Hub from servo"; arm_num "Arm number"; eta_dir "eta direcction"; gamma_dir "gamma direction"; J_T "Inertia Motor+prop"; J_FA "Inertia Forearm"; h "h propeller hub"; Torq_ini "Torque Initial Condition"; Omega_ini "Omega Initial Condition"; init_eta "Initial eta  (rad)"; init_gamma "Initial gamma  (rad)"; omega_n "Servo natural frequency"; xi "Servo damping"; c "Derivative param"
      mask help:
      | This block only accepts arms oriented in x-axis or y-axis: eta and gamma directions can only be [1,0,0] or [0,1,0]
      | Note rotations order is [eta (pan) ,gamma (tilt),0]
      |
      | If Arm number 1 (Forward one)
      | eta_dir=[1,0,0]
      | gamma_dir=[0,1,0]
      |
      | If Arm number 2 or 3 (rear ones)
      | eta_dir=[0,1,0]
      | gamma_dir=[1,0,0]
      mask TypeOptions Rot_sign: Aerodynamics Propeller/Rot_sign | Gyroscopic Moments/Rot_sign
      mask TypeOptions tau: ESC+Motor Dynamcis/tau
      mask TypeOptions arm_hub_pos: Arms Kinematics/Arm_hub_position
      mask TypeOptions arm_axis: Gyroscopic Moments/Arm_axis
      mask TypeOptions arm_num: Arms Kinematics/Arm_number
      mask TypeOptions eta_dir: Arms Kinematics/eta_dir | Gyroscopic Moments/eta_dir
      mask TypeOptions gamma_dir: Arms Kinematics/gamma_dir | Gyroscopic Moments/gamma_dir
      mask TypeOptions J_T: ESC+Motor Dynamcis/J_T | Gyroscopic Moments/J_T
      mask TypeOptions J_FA: Gyroscopic Moments/J_FA
      mask TypeOptions h: Arms Kinematics/h_prop
      mask TypeOptions Torq_ini: Initial_torque/X0
      mask TypeOptions Omega_ini: initial_omega/X0
      mask TypeOptions init_eta: Servos Dynamics/init_eta
      mask TypeOptions omega_n: Servos Dynamics/omega_n
      mask TypeOptions xi: Servos Dynamics/xi
      mask TypeOptions c: Servos Dynamics/derv_param
      mask Display:
      | % fprintf(' Arm number %i \n dynamics',arm_num)
      | 
      | 
      | disp(['{\bf \fontsize{16}',sprintf('Arm number\n\n'),num2str(arm_num),sprintf('\n\n Dynamics '),'}'], 'texmode','on');
  Arm Dynamics1 : Subsystem  AncestorBlock=XXCopter/Arm Dynamics  TreatAsAtomicUnit=on  mask(Arm dynamics, kinematics, forces and moments){Rot_sign=Rotation_sign(2), tau=Tau_motors, arm_hub_pos=l*[-1/2;sqrt(3)/2;0], arm_axis=[0;l_arm;0], arm_num=2, eta_dir=[0;1;0], gamma_dir=[1;0;0], J_T=J_T, J_FA=J_FA, h=h, Torq_ini=Initial_Torques(2), Omega_ini=Initial_Omegas(2), init_eta=0, init_gamma=0, omega_n=35, xi=1.45, c=0.01}
      mask prompts: Rot_sign "Rotation sign"; tau "Tau motors"; arm_hub_pos "Arm Hub position"; arm_axis "Arm Hub from servo"; arm_num "Arm number"; eta_dir "eta direcction"; gamma_dir "gamma direction"; J_T "Inertia Motor+prop"; J_FA "Inertia Forearm"; h "h propeller hub"; Torq_ini "Torque Initial Condition"; Omega_ini "Omega Initial Condition"; init_eta "Initial eta  (rad)"; init_gamma "Initial gamma  (rad)"; omega_n "Servo natural frequency"; xi "Servo damping"; c "Derivative param"
      mask help:
      | This block only accepts arms oriented in x-axis or y-axis: eta and gamma directions can only be [1,0,0] or [0,1,0]
      | Note rotations order is [eta (pan) ,gamma (tilt),0]
      |
      | If Arm number 1 (Forward one)
      | eta_dir=[1,0,0]
      | gamma_dir=[0,1,0]
      |
      | If Arm number 2 or 3 (rear ones)
      | eta_dir=[0,1,0]
      | gamma_dir=[1,0,0]
      mask TypeOptions Rot_sign: Aerodynamics Propeller/Rot_sign | Gyroscopic Moments/Rot_sign
      mask TypeOptions tau: ESC+Motor Dynamcis/tau
      mask TypeOptions arm_hub_pos: Arms Kinematics/Arm_hub_position
      mask TypeOptions arm_axis: Gyroscopic Moments/Arm_axis
      mask TypeOptions arm_num: Arms Kinematics/Arm_number
      mask TypeOptions eta_dir: Arms Kinematics/eta_dir | Gyroscopic Moments/eta_dir
      mask TypeOptions gamma_dir: Arms Kinematics/gamma_dir | Gyroscopic Moments/gamma_dir
      mask TypeOptions J_T: ESC+Motor Dynamcis/J_T | Gyroscopic Moments/J_T
      mask TypeOptions J_FA: Gyroscopic Moments/J_FA
      mask TypeOptions h: Arms Kinematics/h_prop
      mask TypeOptions Torq_ini: Initial_torque/X0
      mask TypeOptions Omega_ini: initial_omega/X0
      mask TypeOptions init_eta: Servos Dynamics/init_eta
      mask TypeOptions omega_n: Servos Dynamics/omega_n
      mask TypeOptions xi: Servos Dynamics/xi
      mask TypeOptions c: Servos Dynamics/derv_param
      mask Display:
      | % fprintf(' Arm number %i \n dynamics',arm_num)
      | 
      | 
      | disp(['{\bf \fontsize{16}',sprintf('Arm number\n\n'),num2str(arm_num),sprintf('\n\n Dynamics '),'}'], 'texmode','on');
  Arm Dynamics2 : Subsystem  AncestorBlock=XXCopter/Arm Dynamics  TreatAsAtomicUnit=on  mask(Arm dynamics, kinematics, forces and moments){Rot_sign=Rotation_sign(3), tau=Tau_motors, arm_hub_pos=l*[-1/2;-sqrt(3)/2;0], arm_axis=[0;-l_arm;0], arm_num=3, eta_dir=[0;1;0], gamma_dir=[1;0;0], J_T=J_T, J_FA=J_FA, h=h, Torq_ini=Initial_Torques(3), Omega_ini=Initial_Omegas(3), init_eta=0, init_gamma=0, omega_n=35, xi=1.45, c=0.01}
      mask prompts: Rot_sign "Rotation sign"; tau "Tau motors"; arm_hub_pos "Arm Hub position"; arm_axis "Arm Hub from servo"; arm_num "Arm number"; eta_dir "eta direcction"; gamma_dir "gamma direction"; J_T "Inertia Motor+prop"; J_FA "Inertia Forearm"; h "h propeller hub"; Torq_ini "Torque Initial Condition"; Omega_ini "Omega Initial Condition"; init_eta "Initial eta  (rad)"; init_gamma "Initial gamma  (rad)"; omega_n "Servo natural frequency"; xi "Servo damping"; c "Derivative param"
      mask help:
      | This block only accepts arms oriented in x-axis or y-axis: eta and gamma directions can only be [1,0,0] or [0,1,0]
      | Note rotations order is [eta (pan) ,gamma (tilt),0]
      |
      | If Arm number 1 (Forward one)
      | eta_dir=[1,0,0]
      | gamma_dir=[0,1,0]
      |
      | If Arm number 2 or 3 (rear ones)
      | eta_dir=[0,1,0]
      | gamma_dir=[1,0,0]
      mask TypeOptions Rot_sign: Aerodynamics Propeller/Rot_sign | Gyroscopic Moments/Rot_sign
      mask TypeOptions tau: ESC+Motor Dynamcis/tau
      mask TypeOptions arm_hub_pos: Arms Kinematics/Arm_hub_position
      mask TypeOptions arm_axis: Gyroscopic Moments/Arm_axis
      mask TypeOptions arm_num: Arms Kinematics/Arm_number
      mask TypeOptions eta_dir: Arms Kinematics/eta_dir | Gyroscopic Moments/eta_dir
      mask TypeOptions gamma_dir: Arms Kinematics/gamma_dir | Gyroscopic Moments/gamma_dir
      mask TypeOptions J_T: ESC+Motor Dynamcis/J_T | Gyroscopic Moments/J_T
      mask TypeOptions J_FA: Gyroscopic Moments/J_FA
      mask TypeOptions h: Arms Kinematics/h_prop
      mask TypeOptions Torq_ini: Initial_torque/X0
      mask TypeOptions Omega_ini: initial_omega/X0
      mask TypeOptions init_eta: Servos Dynamics/init_eta
      mask TypeOptions omega_n: Servos Dynamics/omega_n
      mask TypeOptions xi: Servos Dynamics/xi
      mask TypeOptions c: Servos Dynamics/derv_param
      mask Display:
      | % fprintf(' Arm number %i \n dynamics',arm_num)
      | 
      | 
      | disp(['{\bf \fontsize{16}',sprintf('Arm number\n\n'),num2str(arm_num),sprintf('\n\n Dynamics '),'}'], 'texmode','on');
  Bus Creator : BusCreator  Inputs=3
  Bus Creator1 : BusCreator  Inputs=3
  Comm Angles (deg)1 : InportShadow  Port=2
  Comm Angles (deg)2 : InportShadow  Port=2
  Degrees to Radians1 : simulink_extras/Transformations/Degrees to Radians
  Degrees to Radians2 : simulink_extras/Transformations/Degrees to Radians
  Degrees to Radians3 : simulink_extras/Transformations/Degrees to Radians
  Forces_add : Sum  Inputs=+++
  Initial Omegas1 : InportShadow  Port=3
  Initial Omegas2 : InportShadow  Port=3
  Moments add : Sum  Inputs=+++
  Mux : Mux  Inputs=3
  Mux1 : Mux  Inputs=3
  Selector : Selector  InputPortWidth=3  Indices=[1]
  Selector1 : Selector  InputPortWidth=3  Indices=[1]
  Selector2 : Selector  InputPortWidth=6  Indices=[1,2]
  Selector3 : Selector  InputPortWidth=3  Indices=2
  Selector4 : Selector  InputPortWidth=3  Indices=2
  Selector5 : Selector  InputPortWidth=6  Indices=[3,4]
  Selector6 : Selector  InputPortWidth=3  Indices=3
  Selector7 : Selector  InputPortWidth=3  Indices=3
  Selector8 : Selector  InputPortWidth=6  Indices=[5,6]
  Throttles1 : InportShadow
  Throttles2 : InportShadow
  V_b1 : InportShadow  Port=5
  V_b2 : InportShadow  Port=5
  h_ground1 : InportShadow  Port=6
  h_ground2 : InportShadow  Port=6
  omega_b1 : InportShadow  Port=4
  omega_b2 : InportShadow  Port=4
  Forces : Outport
  Moments : Outport  Port=2
  Omegas : Outport  Port=3
  Omegas_dot : Outport  Port=4
  Arms DCMs : Outport  Port=5
  Angles (rad) : Outport  Port=6
  tag scope: r_p_1=global, r_p_2=global, r_p_3=global
  wires:
  Selector1/1 -> Arm Dynamics/3(Omega_Initial)
  Throttles/1 -> Selector/1
  Initial Omegas/1 -> Selector1/1
  Selector/1 -> Arm Dynamics/1(Throttle [0-1])
  V_b/1 -> Arm Dynamics/6(V_b)
  Forces_add/1 -> Forces/1
  Moments add/1 -> Moments/1
  Mux/1 -> Omegas/1
  Mux1/1 -> Omegas_dot/1
  h_ground/1 -> Arm Dynamics/4(h_ground)
  Arm Dynamics/1(Forces) -> [F_arm1]
  Arm Dynamics/2(Moments) -> [M_arm1]
  Arm Dynamics/3(Omega_out) -> [Omega1]
  Arm Dynamics/4(Omega_dot_out) -> [Omega_dot1]
  [F_arm1] -> Forces_add/1
  [M_arm1] -> Moments add/1
  [Omega_dot1] -> Mux1/1
  [Omega1] -> Mux/1
  omega_b/1 -> Arm Dynamics/5(omega_b)
  [F_arm2] -> Forces_add/2
  [F_arm3] -> Forces_add/3
  [Omega2] -> Mux/2
  [Omega3] -> Mux/3
  [Omega_dot2] -> Mux1/2
  [Omega_dot3] -> Mux1/3
  [M_arm3] -> Moments add/3
  [M_arm2] -> Moments add/2
  Degrees to Radians1/1 -> Arm Dynamics/2(Comm Angles (rad))
  Comm Angles (deg)/1 -> Selector2/1
  Selector2/1 -> Degrees to Radians1/1
  Arm Dynamics/5(T_FaFb) -> [T1_FaFb]  "T_FaFb1"
  Bus Creator/1 -> Arms DCMs/1
  [T1_FaFb] -> Bus Creator/1
  Selector4/1 -> Arm Dynamics1/3(Omega_Initial)
  Throttles1/1 -> Selector3/1
  Initial Omegas1/1 -> Selector4/1
  Selector3/1 -> Arm Dynamics1/1(Throttle [0-1])
  V_b1/1 -> Arm Dynamics1/6(V_b)
  h_ground1/1 -> Arm Dynamics1/4(h_ground)
  Arm Dynamics1/1(Forces) -> [F_arm2]
  Arm Dynamics1/2(Moments) -> [M_arm2]
  Arm Dynamics1/3(Omega_out) -> [Omega2]
  Arm Dynamics1/4(Omega_dot_out) -> [Omega_dot2]
  omega_b1/1 -> Arm Dynamics1/5(omega_b)
  Degrees to Radians2/1 -> Arm Dynamics1/2(Comm Angles (rad))
  Comm Angles (deg)1/1 -> Selector5/1
  Selector5/1 -> Degrees to Radians2/1
  Arm Dynamics1/5(T_FaFb) -> [T2_FaFb]  "T_FaFb2"
  [T2_FaFb] -> Bus Creator/2
  Selector7/1 -> Arm Dynamics2/3(Omega_Initial)
  Throttles2/1 -> Selector6/1
  Initial Omegas2/1 -> Selector7/1
  Selector6/1 -> Arm Dynamics2/1(Throttle [0-1])
  V_b2/1 -> Arm Dynamics2/6(V_b)
  h_ground2/1 -> Arm Dynamics2/4(h_ground)
  Arm Dynamics2/1(Forces) -> [F_arm3]
  Arm Dynamics2/2(Moments) -> [M_arm3]
  Arm Dynamics2/3(Omega_out) -> [Omega3]
  Arm Dynamics2/4(Omega_dot_out) -> [Omega_dot3]
  omega_b2/1 -> Arm Dynamics2/5(omega_b)
  Degrees to Radians3/1 -> Arm Dynamics2/2(Comm Angles (rad))
  Comm Angles (deg)2/1 -> Selector8/1
  Selector8/1 -> Degrees to Radians3/1
  Arm Dynamics2/5(T_FaFb) -> [T3_FaFb]  "T_FaFb3"
  [T3_FaFb] -> Bus Creator/3
  Bus Creator1/1 -> Angles (rad)/1
  [Angles_1] -> Bus Creator1/1
  [Angles_2] -> Bus Creator1/2
  [Angles_3] -> Bus Creator1/3
  Arm Dynamics/6(Angles (rad)) -> [Angles_1]  "Angles Arm 1"
  Arm Dynamics1/6(Angles (rad)) -> [Angles_2]  "Angles Arm 2"
  Arm Dynamics2/6(Angles (rad)) -> [Angles_3]  "Angles Arm 3"
  Arm Dynamics/7(r_p) -> [r_p_1]
  Arm Dynamics1/7(r_p) -> [r_p_2]
  Arm Dynamics2/7(r_p) -> [r_p_3]
